simulink model "Transformations"  (R2014b)
settings: Solver=ode45  StartTime=0.0  StopTime=10.0  RelTol=1e-3
settings Model: Creator=Lei  LastModifiedBy=Lei

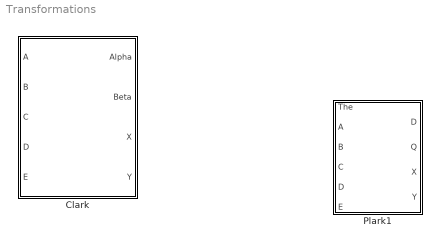
== system Transformations ==
  Clark : Subsystem
  Plark1 : Subsystem

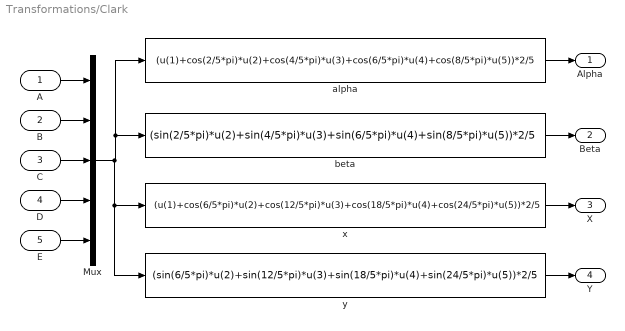
== system Transformations/Clark ==
  A : Inport
  B : Inport  Port=2
  C : Inport  Port=3
  D : Inport  Port=4
  E : Inport  Port=5
  Mux : Mux  Inputs=5
  alpha : Fcn  Expr=(u(1)+cos(2/5*pi)*u(2)+cos(4/5*pi)*u(3)+cos(6/5*pi)*u(4)+cos(8/5*pi)*u(5))*2/5
  beta : Fcn  Expr=(sin(2/5*pi)*u(2)+sin(4/5*pi)*u(3)+sin(6/5*pi)*u(4)+sin(8/5*pi)*u(5))*2/5
  "x " : Fcn  Expr=(u(1)+cos(6/5*pi)*u(2)+cos(12/5*pi)*u(3)+cos(18/5*pi)*u(4)+cos(24/5*pi)*u(5))*2/5
  "y " : Fcn  Expr=(sin(6/5*pi)*u(2)+sin(12/5*pi)*u(3)+sin(18/5*pi)*u(4)+sin(24/5*pi)*u(5))*2/5
  Alpha : Outport
  Beta : Outport  Port=2
  X : Outport  Port=3
  Y : Outport  Port=4
  wires:
  alpha/1 -> Alpha/1
  B/1 -> Mux/2
  C/1 -> Mux/3
  A/1 -> Mux/1
  beta/1 -> Beta/1
  D/1 -> Mux/4
  E/1 -> Mux/5
  Mux/1 -> "x "/1, "y "/1, alpha/1, beta/1
  "x "/1 -> X/1
  "y "/1 -> Y/1

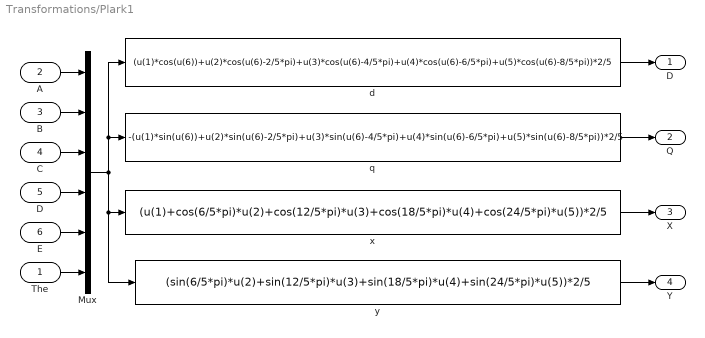
== system Transformations/Plark1 ==
  The : Inport
  A : Inport  Port=2
  B : Inport  Port=3
  C : Inport  Port=4
  D : Inport  Port=5
  E : Inport  Port=6
  Mux : Mux  Inputs=6
  d : Fcn  Expr=(u(1)*cos(u(6))+u(2)*cos(u(6)-2/5*pi)+u(3)*cos(u(6)-4/5*pi)+u(4)*cos(u(6)-6/5*pi)+u(5)*cos(u(6)-8/5*pi))*2/5
  q : Fcn  Expr=-(u(1)*sin(u(6))+u(2)*sin(u(6)-2/5*pi)+u(3)*sin(u(6)-4/5*pi)+u(4)*sin(u(6)-6/5*pi)+u(5)*sin(u(6)-8/5*pi))*2/5
  "x " : Fcn  Expr=(u(1)+cos(6/5*pi)*u(2)+cos(12/5*pi)*u(3)+cos(18/5*pi)*u(4)+cos(24/5*pi)*u(5))*2/5
  "y " : Fcn  Expr=(sin(6/5*pi)*u(2)+sin(12/5*pi)*u(3)+sin(18/5*pi)*u(4)+sin(24/5*pi)*u(5))*2/5
  "D " : Outport
  Q : Outport  Port=2
  X : Outport  Port=3
  Y : Outport  Port=4
  wires:
  d/1 -> "D "/1
  B/1 -> Mux/2
  C/1 -> Mux/3
  A/1 -> Mux/1
  D/1 -> Mux/4
  E/1 -> Mux/5
  The/1 -> Mux/6
  Mux/1 -> q/1, d/1, "y "/1, "x "/1
  q/1 -> Q/1
  "x "/1 -> X/1
  "y "/1 -> Y/1
